simulink subsystem "Path_Planning"  (R2023b)
settings: Solver=VariableStepAuto  StartTime=0.0  StopTime=10.0  RelTol=1e-3
undefined symbols (not defined in the file): Spline_Num_Samples
libraries: simulink x1
settings Model: Creator=FIRSTMentor  LastModifiedBy=FIRSTMentor

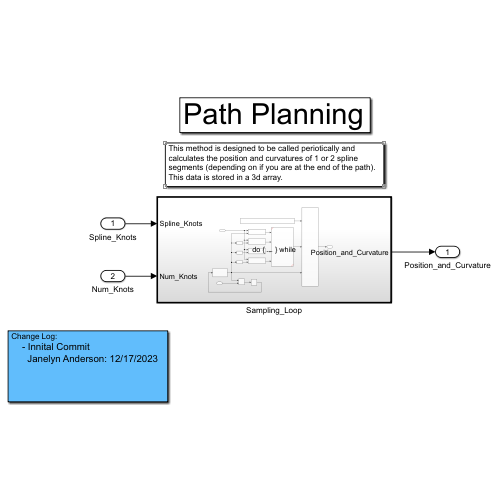
[thumbnail: Simulink's stored preview of the top-level diagram]
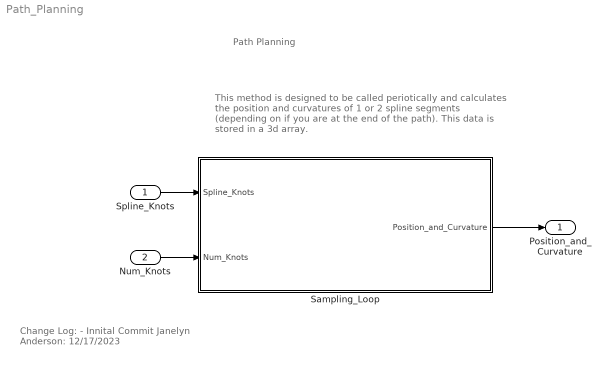
== system Path_Planning ==
  note: This method is designed to be called periotically and calculates the position and curvatures of 1 or 2 spline segments (depending on if you are at the end of the path). This data is stored in a 3d array.
  note: Path Planning
  note: Change Log:
      | - Innital Commit
      | Janelyn Anderson: 12/17/2023
  Spline_Knots : Inport
  Num_Knots : Inport  Port=2
  Sampling_Loop : Subsystem  TreatAsAtomicUnit=on
  Position_and_Curvature : Outport
  wires:
  Spline_Knots/1 -> Sampling_Loop/1(Spline_Knots)
  Num_Knots/1 -> Sampling_Loop/2(Num_Knots)
  Sampling_Loop/1(Position_and_Curvature) -> Position_and_Curvature/1

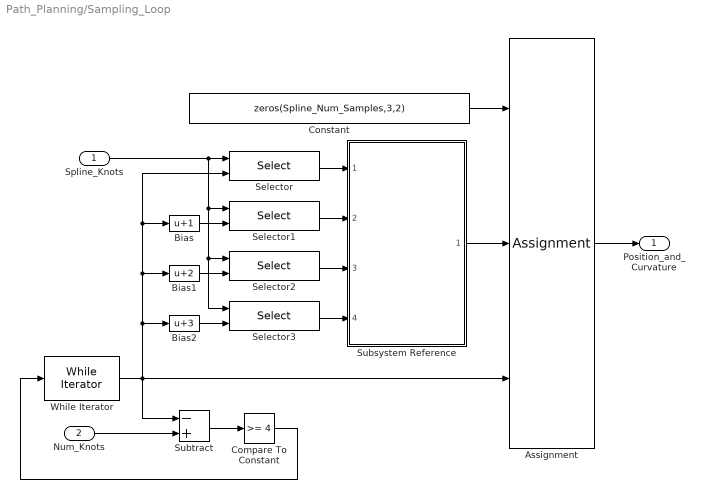
== system Path_Planning/Sampling_Loop ==
  Spline_Knots : Inport
  Num_Knots : Inport  Port=2
  Assignment : Assignment  NumberOfDimensions=3  DiagnosticForDimensions=Warning  IndexOptions=Assign all,Assign all,Index vector (port)  Indices=1,1,1  OutputSizes=1,1,1
  Bias : Bias  Bias=1  SaturateOnIntegerOverflow=off
  Bias1 : Bias  Bias=2  SaturateOnIntegerOverflow=off
  Bias2 : Bias  Bias=3  SaturateOnIntegerOverflow=off
  Compare To Constant : simulink/Logic and Bit Operations/Compare To Constant  relop=>=  const=4  OutDataTypeStr=boolean
  Constant : Constant  Value=zeros(Spline_Num_Samples,3,2)  VectorParams1D=off
  Selector{,1..3} (4 alike) : Selector  NumberOfDimensions=2  InputPortWidth=3  IndexOptions=Index vector (port),Select all  Indices=[1 3],1  OutputSizes=1,1
  Subsystem Reference : Subsystem  ReferencedSubsystem=Sample_Catmull_Rom_Pos_And_Curve
  Subtract : Sum  Inputs=-+
  While Iterator : WhileIterator  MaxIters=2  WhileBlockType=do-while  ShowIterationPort=on
  Position_and_Curvature : Outport
  wires:
  While Iterator/1 -> Subtract/1, Assignment/3, Bias2/1, Bias1/1, Bias/1, Selector/2
  Spline_Knots/1 -> Selector3/1, Selector2/1, Selector1/1, Selector/1
  Selector/1 -> Subsystem Reference/1
  Selector3/1 -> Subsystem Reference/4
  Selector2/1 -> Subsystem Reference/3
  Selector1/1 -> Subsystem Reference/2
  Bias2/1 -> Selector3/2
  Bias1/1 -> Selector2/2
  Bias/1 -> Selector1/2
  Subsystem Reference/1 -> Assignment/2
  Assignment/1 -> Position_and_Curvature/1
  Constant/1 -> Assignment/1
  Num_Knots/1 -> Subtract/2
  Subtract/1 -> Compare To Constant/1
  Compare To Constant/1 -> While Iterator/1
